simulink model "tutorial03_first_order"  (R2025a)
settings: Solver=VariableStepAuto  StartTime=0.0  StopTime=10.0  RelTol=1e-3
settings Model: Creator=xing2  LastModifiedBy=xing2

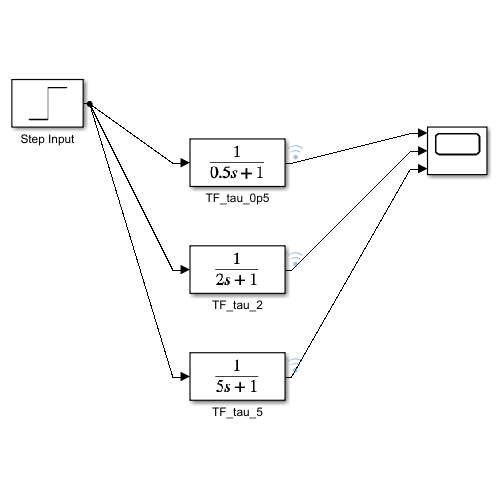
[thumbnail: Simulink's stored preview of the top-level diagram]
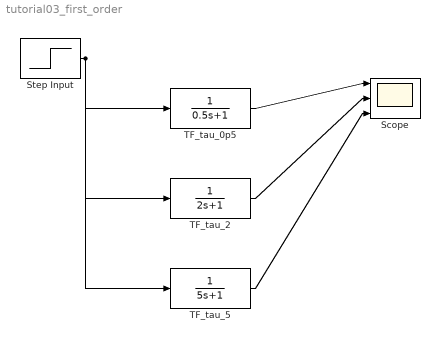
== system tutorial03_first_order ==
  Scope : Scope  NumInputPorts=3
  Step Input : Step  SampleTime=0
  TF_tau_0p5 : TransferFcn  Denominator=[0.5 1]
  TF_tau_2 : TransferFcn  Denominator=[2 1]
  TF_tau_5 : TransferFcn  Denominator=[5 1]
  wires:
  Step Input/1 -> TF_tau_0p5/1, TF_tau_2/1, TF_tau_5/1
  TF_tau_0p5/1 -> Scope/1
  TF_tau_2/1 -> Scope/2
  TF_tau_5/1 -> Scope/3
